simulink model "rig_real_time_template_2023"  (R2023b)
settings: Solver=ode1  StartTime=0.0  StopTime=60  RelTol=1e-3  EnableMultiTasking=on
values from neighbouring files (symbols this model uses):
  den = cell2mat(HY3_N1_D.denominator)    [Question_3.m]    (also in threeDiskOscillator_RIG_template_2023.m)
  den2 = cell2mat(HY3_N2_D.denominator)    [Question_3.m]    (also in threeDiskOscillator.m; threeDiskOscillator_RIG_template_2023.m)
  num_HU2_N1_D = cell2mat(HU2_N1_D.numerator)    [Question_3.m]    (also in threeDiskOscillator.m; threeDiskOscillator_RIG_template_2023.m)
  num_HY1_N1_D = cell2mat(HY1_N1_D.numerator)    [Question_3.m]    (also in threeDiskOscillator.m; threeDiskOscillator_RIG_template_2023.m)
  num_HY2_N1_D = cell2mat(HY2_N1_D.numerator)    [Question_3.m]    (also in threeDiskOscillator.m; threeDiskOscillator_RIG_template_2023.m)
  num_HY2_N2_D = cell2mat(HY2_N2_D.numerator)    [Question_3.m]    (also in threeDiskOscillator.m; threeDiskOscillator_RIG_template_2023.m)
  num_HY3_N1_D = cell2mat(HY3_N1_D.numerator)    [Question_3.m]    (also in threeDiskOscillator.m; threeDiskOscillator_RIG_template_2023.m)
  num_HY3_N2_D = cell2mat(HY3_N2_D.numerator)    [Question_3.m]    (also in threeDiskOscillator.m; threeDiskOscillator_RIG_template_2023.m)
settings Model: SimulationMode=external  ExtModeTrigDuration=75001  Creator=Dro  LastModifiedBy=giova
settings SolverCC: AlgebraicLoopSolver=TrustRegion
settings DataIOCC: LimitDataPoints=on  SaveFormat=Array  ReturnWorkspaceOutputs=off  SignalLoggingName=sigsOut
settings OptimizationCC: ExpressionDepthLimit=2147483647  InitFltsAndDblsToZero=on
settings DebuggingCC: SaveWithParameterizedLinksMsg=none  UnderspecifiedInitializationDetection=Classic  MergeDetectMultiDrivingBlocksExec=none  SignalResolutionControl=TryResolveAllWithWarning  MultiTaskDSMMsg=warning  MultiTaskCondExecSysMsg=none  FcnCallInpInsideContextMsg=warning  UnconnectedInputMsg=warning  UnconnectedOutputMsg=warning  UnconnectedLineMsg=warning  StateNameClashWarn=warning  SFUnexpectedBacktrackingDiag=warning  SFNoUnconditionalDefaultTransitionDiag=warning  SFExecutionAtInitializationDiag=none  ArithmeticOperatorsInVariantConditions=warning
settings HardwareCC: ProdBitPerLong=64  ProdHWDeviceType=Intel->x86-64 (Linux 64)
settings ModelReferenceCC: EnableRefExpFcnMdlSchedulingChecks=on  PropagateSignalLabelsOutOfModel=off
settings SFSimCC: SimUseLocalCustomCode=off  CustomCodeUndefinedFunction=UseInterfaceOnly
settings RTWCC: Description=Simulink Desktop Real-Time  SystemTargetFile=sldrt.tlc  TemplateMakefile=sldrt.tmf  RTWUseLocalCustomCode=off  RTWCompilerOptimization=on
settings CodeAppCC: MaxIdLength=95  StateflowObjectComments=on
settings SimulinkDesktopRealTimeCC: TargetLibSuffix=_sldrt.a  TargetPreCompLibLocation=C:\Program Files\MATLAB\R2023b\toolbox\sldrt\lib\win64  TargetLangStandard=C89/C90 (ANSI)
settings ConfigComp: CovMetricSettings=dw  CovSaveCumulativeToWorkspaceVar=on  CovSaveSingleToWorkspaceVar=on  CovExternalEMLEnable=off

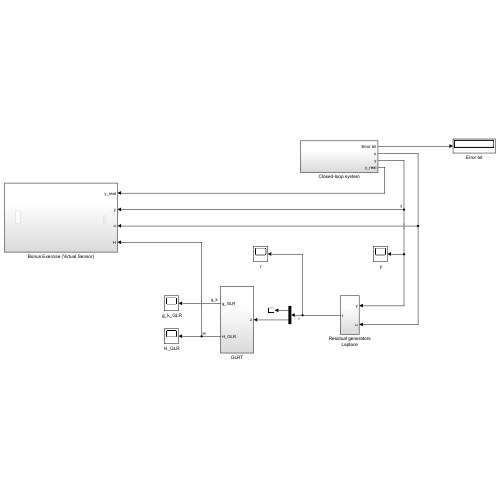
[thumbnail: Simulink's stored preview of the top-level diagram]
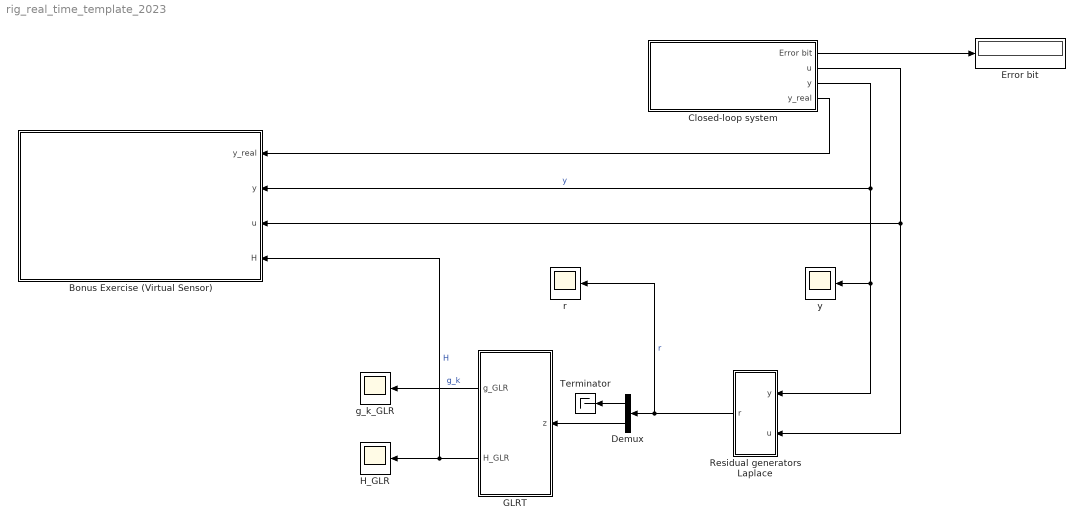
== system rig_real_time_template_2023 ==
  " H_GLR" : Scope
  " g_k_GLR" : Scope
  " r" : Scope
  " y" : Scope
  Bonus Exercise (Virtual Sensor) : Subsystem
  Closed-loop system : Subsystem
  Demux : Demux  Outputs=2
  "Error bit " : Display
  GLRT : Subsystem
  Residual generators Laplace : Subsystem
  Terminator : Terminator
  wires:
  Closed-loop system/2(u) -> Residual generators Laplace/2(u), Bonus Exercise (Virtual Sensor)/3(u)
  Closed-loop system/1(Error bit) -> "Error bit "/1
  Residual generators Laplace/1(r) -> Demux/1, " r"/1  "r"
  Closed-loop system/3(y) -> Residual generators Laplace/1(y), " y"/1, Bonus Exercise (Virtual Sensor)/2(y)  "y"
  GLRT/1(g_GLR) -> " g_k_GLR"/1  "g_k"
  GLRT/2(H_GLR) -> Bonus Exercise (Virtual Sensor)/4(H), " H_GLR"/1  "H"
  Closed-loop system/4(y_real) -> Bonus Exercise (Virtual Sensor)/1(y_real)
  Demux/2 -> GLRT/1(z)
  Demux/1 -> Terminator/1

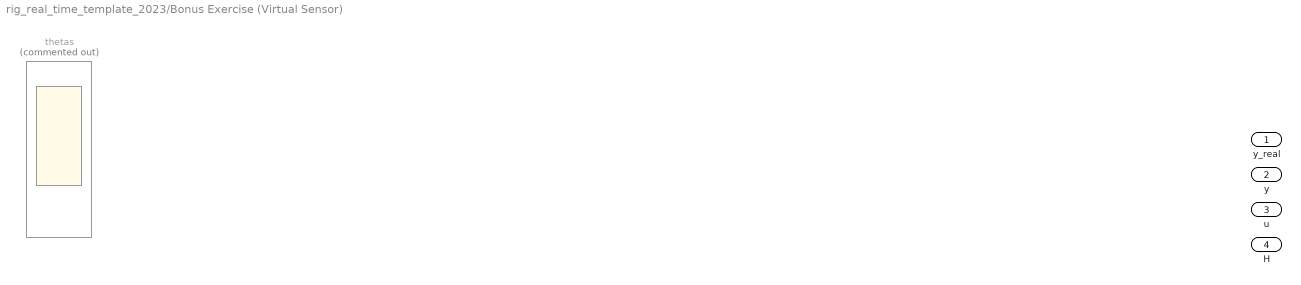
== system rig_real_time_template_2023/Bonus Exercise (Virtual Sensor) ==
  y_real : Inport
  y : Inport  Port=2
  u : Inport  Port=3
  H : Inport  Port=4
  thetas : Scope  Commented=on  NumInputPorts=3

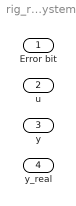
== system rig_real_time_template_2023/Closed-loop system ==
  Error bit : Outport  VectorParamsAs1DForOutWhenUnconnected=off
  u : Outport  Port=2  VectorParamsAs1DForOutWhenUnconnected=off
  y : Outport  Port=3  VectorParamsAs1DForOutWhenUnconnected=off
  y_real : Outport  Port=4  VectorParamsAs1DForOutWhenUnconnected=off

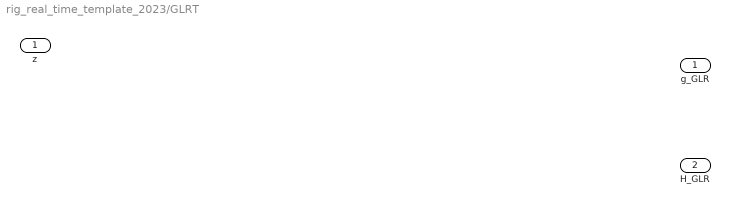
== system rig_real_time_template_2023/GLRT ==
  z : Inport
  g_GLR : Outport  VectorParamsAs1DForOutWhenUnconnected=off
  H_GLR : Outport  Port=2  VectorParamsAs1DForOutWhenUnconnected=off

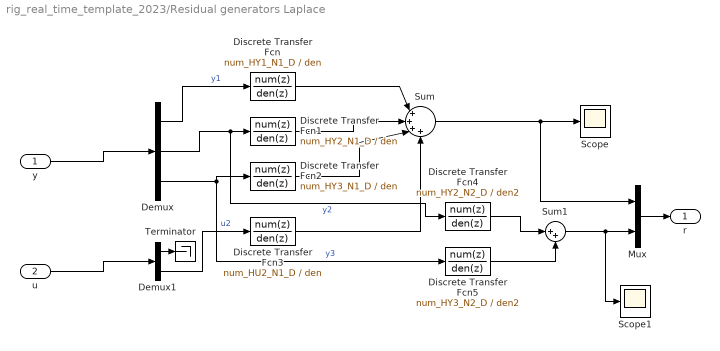
== system rig_real_time_template_2023/Residual generators Laplace ==
  y : Inport
  u : Inport  Port=2
  Demux : Demux  Outputs=3
  Demux1 : Demux  Outputs=2
  Discrete Transfer Fcn : DiscreteTransferFcn  Numerator=num_HY1_N1_D  Denominator=den
  Discrete Transfer Fcn1 : DiscreteTransferFcn  Numerator=num_HY2_N1_D  Denominator=den
  Discrete Transfer Fcn2 : DiscreteTransferFcn  Numerator=num_HY3_N1_D  Denominator=den
  Discrete Transfer Fcn3 : DiscreteTransferFcn  Numerator=num_HU2_N1_D  Denominator=den
  Discrete Transfer Fcn4 : DiscreteTransferFcn  Numerator=num_HY2_N2_D  Denominator=den2
  Discrete Transfer Fcn5 : DiscreteTransferFcn  Numerator=num_HY3_N2_D  Denominator=den2
  Mux : Mux  Inputs=2
  Scope : Scope
  Scope1 : Scope
  Sum : Sum  Inputs=|++++
  Sum1 : Sum  Inputs=|++
  Terminator : Terminator
  r : Outport  VectorParamsAs1DForOutWhenUnconnected=off
  wires:
  Discrete Transfer Fcn5/1 -> Sum1/2
  Discrete Transfer Fcn/1 -> Sum/1
  Discrete Transfer Fcn1/1 -> Sum/2
  Discrete Transfer Fcn3/1 -> Sum/4
  Demux1/2 -> Discrete Transfer Fcn3/1  "u2"
  Discrete Transfer Fcn2/1 -> Sum/3
  Demux1/1 -> Terminator/1
  Sum1/1 -> Scope1/1, Mux/2
  Mux/1 -> r/1
  Sum/1 -> Scope/1, Mux/1
  Demux/3 -> Discrete Transfer Fcn5/1, Discrete Transfer Fcn2/1  "y3"
  Discrete Transfer Fcn4/1 -> Sum1/1
  Demux/2 -> Discrete Transfer Fcn4/1, Discrete Transfer Fcn1/1  "y2"
  Demux/1 -> Discrete Transfer Fcn/1  "y1"
  y/1 -> Demux/1
  u/1 -> Demux1/1
